simulink model "AC_DC_BUCK_2022b"  (R2022b)
settings: Solver=VariableStepAuto  StartTime=0.0  StopTime=3  RelTol=1e-3
libraries: spsSeriesRLCBranchLib x16, spsIdealSwitchLib x9, gmp_peripheral_utilities x6, spsVoltageMeasurementLib x6, spsSecondOrderFilterLib x5, spsControlledVoltageSourceLib x3, spsCurrentMeasurementLib x2, gmp_sil_core_pack x1, spspowerguiLib x1
(part 1 of 2)
settings Model: SimulationMode=accelerator  Creator=javnson  LastModifiedBy=javnson
settings DataIOCC: ReturnWorkspaceOutputs=off
settings OptimizationCC: ReuseModelBlockBuffer=on
settings RTWCC: GPUComputeCapability=5.0

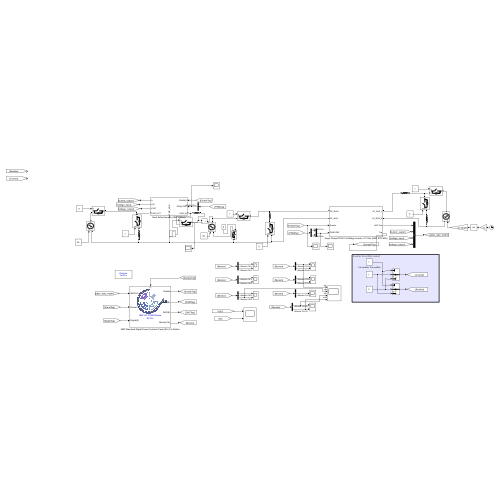
[thumbnail: Simulink's stored preview of the top-level diagram]
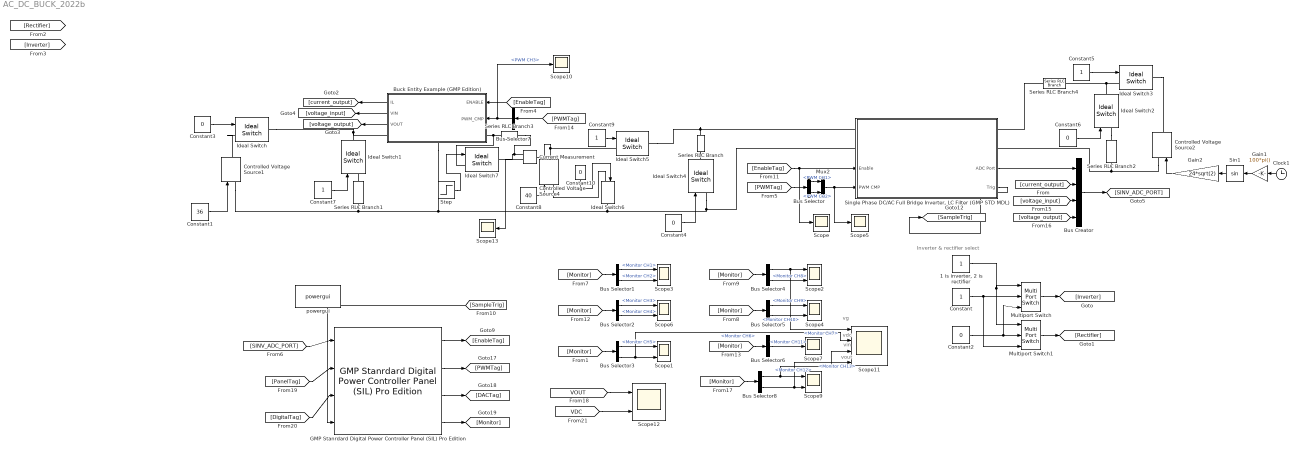
== system AC_DC_BUCK_2022b ==
  note: vout
  note: vin
  note: vg
  note: vdc
  note: Inverter & rectifier select
  "1 is inverter, 2 is rectifier" : Constant
  Buck Entity Example (GMP Edition) : Subsystem  mask{Cin=680e-6, Cout=680e-6, L=50e-6, RL=1e-3, RCin=0.1, RCout=100e-6, Cout2=680e-6, RCout2=1e-4, Voadc_bias=0, Voadc_fs=120, ADC_RES=16, Viadc_fs=120, Viadc_bias=0, Iladc_fs=60, Iadc_bias=30, fswitch=20e3, CMP_MAX=4200-1, DB_UP=100, DB_DW=100, Rds_on=0.02, Lon=0, Rd=0.01, Vf=0.3, Rs=1e5, Cs=inf}
      settings: PortSchema="{\"entries\":[{\"content\":{\"sides\":[{\"content\":{\"connectorIds\":[\"In1\",\"In2\",\"LConn1\"]},\"type\":\"ConnectorPlacement.EquallySpacedRectSide\",\"uuid\":\"3dc1f0aa-256b-4eee-9ab4-ff52cb056450\"},{\"content\":{\"connectorIds\":[\"Out1\",\"Out2\",\"Out3\",\"RConn1\"],\"side\":\"RIGHT\"},\"type\":\"ConnectorPlacement.EquallySpacedRectSide\",\"uuid\":\"c182f68c-961e-48e9-b450-8a2d07cca989\"},{\"content\":{\"connectorIds\":[],\"side\":\"TOP\"},\"type\":\"ConnectorPlacement.EquallySpacedRectSide\",\"uuid\":\"77cafdf0-ba99-4ec6-a003-27712a389068\"},{\"content\":{\"connectorIds\":[\"RConn2\"],\"side\":\"BOTTOM\"},\"type\":\"ConnectorPlacement.EquallySpacedRectSide\",\"uuid\":\"1cb5a4dc-5d4b-4bbe-a9bd-2c66268ddaed\"}]},\"type\":\"ConnectorPlacement.EquallySpacedConnector\",\"uuid\":\"ec8c1d3d-5436-4386-91dc-89cedd685bc0\"}],\"packageUris\":[\"http://schema.mathworks.com/mf0/Connector/R2020b\"],\"version\":\"1.0\"}"
      mask DialogControl Container4 Prompt: Main Circuit
      mask DialogControl Control2 Prompt: Input port Capacitor, unit F
      mask DialogControl Control3 Prompt: Ouput port Capacitor, unit F
      mask DialogControl Control4 Prompt: Filter Inductor, unit H
      mask DialogControl Container6 Prompt: Other Parameters
      mask DialogControl Control5 Prompt: Resistance of Inductor, unit Ohm
      mask DialogControl Control9 Prompt: Resistance of input Capacitor, unit Ohm
      mask DialogControl Control6 Prompt: Resistance of output Capacitor, unit Ohm
      mask DialogControl Control7 Prompt: Low resistance output Capacitor branch, Capacitor, unit F
      mask DialogControl Control8 Prompt: Low resistance output capacitor branch, resistance of capacitor, unit Ohm
      mask DialogControl Container5 Prompt: Sensor
      mask DialogControl Control15 Prompt: Output Voltage ADC, Bias Voltage, unit V
      mask DialogControl Control14 Prompt: Output Voltage ADC, Full Scale Voltage, unit V
      mask DialogControl Control10 Prompt: ADC resolution, bits
      mask DialogControl Control11 Prompt: Input Voltage ADC, Full Scale Voltage, unit V
      mask DialogControl Control12 Prompt: Input Voltage ADC, Bias Voltage, unit V
      mask DialogControl Control13 Prompt: Indctor Current ADC, Full Scale, unit A
      mask DialogControl Control16 Prompt: Inductor Current ADC, Bias Current, unit A
      mask DialogControl Container7 Prompt: PWM Modulator
      mask DialogControl Control17 Prompt: PWM frequency, unit Hz
      mask DialogControl Control18 Prompt: Full Scale PWM Compare value
      mask DialogControl Control19 Prompt: Deadband Setting
      mask DialogControl Container8 Prompt: MOSFET
      mask DialogControl Control20 Prompt: Rds(on), unit Ohm
      mask DialogControl Control21 Prompt: Internal diode inductance, unit H
      mask DialogControl Control22 Prompt: Internal diode resistance Rd, unit Ohm
      mask DialogControl Control23 Prompt: Internal diode forward voltage Vf, unit V
      mask DialogControl Control24 Prompt: Snubber resistance Rs, unit Ohm
      mask DialogControl Control25 Prompt: Snubber Capacitance Cs, unit F
  Bus Creator : BusCreator  Inputs=4
  Bus Selector : BusSelector  OutputSignals=PWM CH1,PWM CH2
  Bus Selector1 : BusSelector  OutputSignals=Monitor CH1,Monitor CH2
  Bus Selector2 : BusSelector  OutputSignals=Monitor CH3,Monitor CH4
  Bus Selector3 : BusSelector  OutputSignals=Monitor CH5,Monitor CH6
  Bus Selector4 : BusSelector  OutputSignals=Monitor CH7,Monitor CH8
  Bus Selector5 : BusSelector  OutputSignals=Monitor CH9,Monitor CH10
  Bus Selector6 : BusSelector  OutputSignals=Monitor CH11
  Bus Selector7 : BusSelector  OutputSignals=PWM CH3
  Bus Selector8 : BusSelector  OutputSignals=Monitor CH12,Monitor CH13
  Clock1 : Clock
  Constant{,5,7,9} (4 alike) : Constant
  Constant1 : Constant  Value=36
  Constant{2..4,6,10} (5 alike) : Constant  Value=0
  Constant8 : Constant  Value=40
  Controlled Voltage Source1 : spsControlledVoltageSourceLib/Controlled Voltage Source  Initialize=on  Source_Type=AC  Amplitude=0  Phase=0  Frequency=0  Measurements=None
  Controlled Voltage Source2 : spsControlledVoltageSourceLib/Controlled Voltage Source  Initialize=on  Source_Type=AC  Amplitude=0  Phase=0  Frequency=0  Measurements=None
  Controlled Voltage Source4 : spsControlledVoltageSourceLib/Controlled Voltage Source  Initialize=on  Source_Type=AC  Amplitude=0  Phase=0  Frequency=0  Measurements=None
  Current Measurement : spsCurrentMeasurementLib/Current Measurement  PhasorSimulation=off  OutputType=Complex  PSBequivalent=0
  GMP Stanrdard Digital Power Controller Panel (SIL) Pro Edition : gmp_sil_core_pack/GMP Stanrdard Digital Power Controller Panel (SIL) Pro Edition
      settings: SourceProductName=GMP SIL Core Utilities
  Gain1 : Gain  Gain=100*pi()
  Gain2 : Gain  Gain=24*sqrt(2)
  Ideal Switch{,1..7} (8 alike) : spsIdealSwitchLib/Ideal Switch  Ron=0.001  Lon=0  IC=0  Rs=1e5  Cs=inf  Measurements=off
  Multiport Switch : MultiPortSwitch  Inputs=2  SaturateOnIntegerOverflow=off  InputSameDT=off
  Multiport Switch1 : MultiPortSwitch  Inputs=2  SaturateOnIntegerOverflow=off  InputSameDT=off
  Mux2 : Mux  Inputs=2
  Scope{,5,7,10,13} (5 alike) : Scope
  Scope{1..4,6,9,12} (7 alike) : Scope  NumInputPorts=2
  Scope11 : Scope  NumInputPorts=4
  Series RLC Branch : spsSeriesRLCBranchLib/Series RLC Branch  LConnTagsString=__new0  RConnTagsString=__new0  BranchType=R  Resistance=100  Inductance=1e-3  SetiL0=off  InitialCurrent=0  Capacitance=1e-6  Setx0=off  InitialVoltage=0  Measurements=None
  Series RLC Branch1 : spsSeriesRLCBranchLib/Series RLC Branch  LConnTagsString=__new0  RConnTagsString=__new0  BranchType=R  Resistance=200  Inductance=1e-3  SetiL0=off  InitialCurrent=0  Capacitance=1e-6  Setx0=off  InitialVoltage=0  Measurements=None
  Series RLC Branch2 : spsSeriesRLCBranchLib/Series RLC Branch  LConnTagsString=__new0  RConnTagsString=__new0  BranchType=R  Resistance=18  Inductance=1e-3  SetiL0=off  InitialCurrent=0  Capacitance=1e-6  Setx0=off  InitialVoltage=0  Measurements=None
  Series RLC Branch3 : spsSeriesRLCBranchLib/Series RLC Branch  LConnTagsString=__new0  RConnTagsString=__new0  BranchType=R  Resistance=100  Inductance=1e-3  SetiL0=off  InitialCurrent=0  Capacitance=1e-6  Setx0=off  InitialVoltage=0  Measurements=None
  Series RLC Branch4 : spsSeriesRLCBranchLib/Series RLC Branch  LConnTagsString=__new0  RConnTagsString=__new0  BranchType=R  Resistance=2  Inductance=1e-3  SetiL0=off  InitialCurrent=0  Capacitance=1e-6  Setx0=off  InitialVoltage=0  Measurements=None
  Sin1 : Trigonometry
  "Single Phase DC/AC Full Bridge Inverter, LC Filter (GMP STD MDL)" : Subsystem  mask(Standard Single Phase DC/AC inverter / rectifier){R_mosfet_on=4.6e-3, Lon=0, Rd=0.01, Vf=0.5, Rs=1e5, Cs=inf, ACF_L=680e-6*2, ACF_L_ESR=0.05, ACF_C=10e-6, ACF_C_ESR=0.02, ACF_C_EPR=100e3, DC_CAP=680e-6, DC_CAP_ESR=0.05, DC_CAP_EPR=10e3, fswitch=20e3, CMP_MAX=4200-1, Deadband_Upper=80, Deadband_Lower=80, phase_shift=0, ADC_Resolution=12, DC_Voltage_Gain=2.2 / 202.2, DC_VOLTAGE_ADC_REFERENCE=2.5, DC_VOLTAGE_ADC_BIAS=0.9966, DC_VOLTAGE_ADC_CUT_FREQ=1.5e3, DC_BUS_CURRENT_SENSOR_R=0.005, DC_Current_Gain=20, DC_CURRENT_ADC_REFERENCE=2.5, DC_CURRENT_ADC_BIAS=0.9, DC_CURRENT_ADC_CUT_FREQ=1.5e3, AC_Voltage_Gain=2.2 / 202.2, AC_VOLTAGE_ADC_REFERENCE=2.5, AC_VOLTAGE_ADC_BIAS=0.9966, AC_VOLTAGE_ADC_CUT_FREQ=1.5e3, AC_Current_Gain=0.005 * 20, AC_CURRENT_ADC_REFERENCE=2.5, AC_CURRENT_ADC_BIAS=0.9, AC_CURRENT_ADC_INIT=0, CAP_CURRENT_SENSOR_R=0.005, CAP_Current_Gain=20, CAP_CURRENT_ADC_REFERENCE=2.5, CAP_CURRENT_ADC_BIAS=0.9, CAP_CURRENT_ADC_CUT_FREQ=1.5e3, GRID_CURRENT_SENSOR_R=0.005, Grid_Current_Gain=20, GRID_CURRENT_ADC_REFERENCE=2.5, GRID_CURRENT_ADC_BIAS=0.9, GRID_CURRENT_ADC_CUT_FREQ=1.5e3}
      mask prompts: ADC_Resolution "ADC_BIT:"; DC_Voltage_Gain "ADC_GAIN:"; DC_VOLTAGE_ADC_REFERENCE "ADC_REFERENCE:"; DC_VOLTAGE_ADC_BIAS "ADC_BIAS:"; DC_VOLTAGE_ADC_CUT_FREQ "cut_frequency:"; DC_Current_Gain "ADC_GAIN:"; DC_CURRENT_ADC_REFERENCE "ADC_REFERENCE:"; DC_CURRENT_ADC_BIAS "ADC_BIAS:"; DC_CURRENT_ADC_CUT_FREQ "ADC_FILTER:"; AC_Voltage_Gain "ADC_GAIN:"; AC_VOLTAGE_ADC_REFERENCE "ADC_REFERENCE:"; AC_VOLTAGE_ADC_BIAS "ADC_BIAS:"; AC_VOLTAGE_ADC_CUT_FREQ "cut_frequency:"; AC_Current_Gain "ADC_GAIN:"; AC_CURRENT_ADC_REFERENCE "ADC_REFERENCE:"; AC_CURRENT_ADC_BIAS "ADC_BIAS:"; AC_CURRENT_ADC_INIT "ADC_INIT:"; CAP_CURRENT_SENSOR_R "CAP_BUS_CURRENT_SENSOR_R:"; CAP_Current_Gain "ADC_GAIN:"; CAP_CURRENT_ADC_REFERENCE "ADC_REFERENCE:"; CAP_CURRENT_ADC_BIAS "ADC_BIAS:"; CAP_CURRENT_ADC_CUT_FREQ "ADC_FILTER:"; GRID_CURRENT_SENSOR_R "DC_BUS_CURRENT_SENSOR_R:"; Grid_Current_Gain "ADC_GAIN:"; GRID_CURRENT_ADC_REFERENCE "ADC_REFERENCE:"; GRID_CURRENT_ADC_BIAS "ADC_BIAS:"; GRID_CURRENT_ADC_CUT_FREQ "ADC_FILTER:"
      mask help: This module takes the inverter direction as the positive direction.
      settings: PortSchema="{\"entries\":[{\"content\":{\"sides\":[{\"content\":{\"connectorIds\":[\"LConn1\",\"LConn2\",\"In1\",\"In2\"]},\"type\":\"ConnectorPlacement.EquallySpacedRectSide\",\"uuid\":\"0e3e6e75-5e1a-455b-8a22-c69d0a4261ca\"},{\"content\":{\"connectorIds\":[\"RConn1\",\"RConn2\",\"Out1\",\"Out2\"],\"side\":\"RIGHT\"},\"type\":\"ConnectorPlacement.EquallySpacedRectSide\",\"uuid\":\"20326781-9238-4fea-80fd-ba96906d5d3f\"},{\"content\":{\"side\":\"TOP\"},\"type\":\"ConnectorPlacement.EquallySpacedRectSide\",\"uuid\":\"9e3289d3-0bee-4337-807b-c293a46cda9c\"}]},\"type\":\"ConnectorPlacement.EquallySpacedConnector\",\"uuid\":\"56bb35ad-d602-4874-b9bf-b95a81ef662c\"}],\"packageUris\":[\"http://schema.mathworks.com/mf0/Connector/R2020b\"],\"version\":\"1.0\"}"
      mask DialogControl ParameterGroupVar Prompt: 参数
      mask DialogControl Container4 Prompt: Component Parameters
      mask DialogControl Container7 Prompt: MOSFET
      mask DialogControl Control2 Prompt: Rds(on), unit Ohm
      mask DialogControl Control3 Prompt: Internal diode inducctance, unit H
      mask DialogControl Control4 Prompt: Internal diode resistance Rd, unit Ohm
      mask DialogControl Control5 Prompt: Internal diode forward voltage Vf, unit V
      mask DialogControl Control6 Prompt: Snubber resistance Rs, unit ohm
      mask DialogControl Control7 Prompt: Snubber Capacitance Cs, unit F
      mask DialogControl Container8 Prompt: LC Filter
      mask DialogControl Container20 Prompt: Filter Inductor
      mask DialogControl Control8 Prompt: AC Bus Filter Inductor (H)
      mask DialogControl Control42 Prompt: AC Bus Filter Inductor, ESR (Ohm)
      mask DialogControl Container21 Prompt: Filter Capcitor
      mask DialogControl Control43 Prompt: AC Bus Filter Capacitor (F)
      mask DialogControl Control44 Prompt: AC Bus Filter Capacitor, ESR (Ohm)
      mask DialogControl Control45 Prompt: AC Bus Filter Capacitor, EPR (Ohm)
      mask DialogControl Container22 Prompt: DC Bus Capacitor
      mask DialogControl Control46 Prompt: DC Bus Capacitor (F)
      mask DialogControl Control47 Prompt: DC Bus Capacitor, ESR (Ohm)
      mask DialogControl Control48 Prompt: DC Bus Capacitor, EPR (Ohm)
      mask DialogControl Container5 Prompt: PWM Parameers
      mask DialogControl Control9 Prompt: PWM Frequency (Hz):
      mask DialogControl Control10 Prompt: Full Scale PWM Compare value:
      mask DialogControl Control11 Prompt: (whole period is 2 * CMP_MAX ticks)
      mask DialogControl Control12 Prompt: Deadband Range Set (CMP Value):
      mask DialogControl Control13 Prompt: Single side deadband time: DEADBAND_CMP/2/CMP_MAX/fswitch
      mask DialogControl Control14 Prompt: Initial Phase Shift, unit rad
      mask DialogControl Container6 Prompt: ADC Parameters
      mask DialogControl Container14 Prompt: ADC Device
      mask DialogControl Control15 Prompt: ADC resolution:
      mask DialogControl Container15 Prompt: DC Side Voltage Sensor
      mask DialogControl Control16 Prompt: ADC Voltage Gain (Scale Factor):
      mask DialogControl Control17 Prompt: ADC reference Voltage(V)
      mask DialogControl Control18 Prompt: ADC Bias Voltage(V)
      mask DialogControl Control19 Prompt: Voltage Filter cut frequency (Hz):
      mask DialogControl Control20 Prompt: Generally, this value less than switch frequency / 10, greater than motor normal frequency * 3
      mask DialogControl Container16 Prompt: DC Side Current Sensor
      mask DialogControl Control26 Prompt: DC Bus Current Sensor Resistance
      mask DialogControl Control34 Prompt: ADC Current Gain (Scale Factor):
      mask DialogControl Control27 Prompt: ADC reference Voltage(V), ADC full scale current (when gain = 1)
      mask DialogControl Control28 Prompt: ADC Bias Current(A)
      mask DialogControl Control35 Prompt: Voltage Filter cut frequency (Hz):
      mask DialogControl Control36 Prompt: Generally, this value less than switch frequency / 10, greater than motor normal frequency * 3
      mask DialogControl Container17 Prompt: AC Side Voltage Sensor
      mask DialogControl Control16_copy Prompt: ADC Voltage Gain (Scale Factor):
      mask DialogControl Control17_copy Prompt: ADC reference Voltage(V)
      mask DialogControl Control18_copy Prompt: ADC Bias Voltage(V)
      mask DialogControl Control19_copy Prompt: Voltage Filter cut frequency (Hz):
      mask DialogControl Control20_copy Prompt: Generally, this value less than switch frequency / 10, greater than motor normal frequency * 3
      mask DialogControl Container18 Prompt: AC Side Current Sensor
      mask DialogControl Control26_copy Prompt: ADC Current Gain (Scale Factor):
      mask DialogControl Control27_copy Prompt: ADC reference Current(A), ADC full scale current (when gain = 1)
      mask DialogControl Control28_copy Prompt: ADC Bias Current(A)
      mask DialogControl Control29_copy Prompt: ADC initial Current Output(A)
      mask DialogControl Container19 Prompt: Capcitor Current Sensor
      mask DialogControl Control26_copy_copy Prompt: Filter Capacitor Current Sensor Resistance
      mask DialogControl Control34_copy Prompt: ADC Current Gain (Scale Factor):
      mask DialogControl Control27_copy_copy Prompt: ADC reference Voltage(V), ADC full scale current (when gain = 1)
      mask DialogControl Control28_copy_copy Prompt: ADC Bias Current(V)
      mask DialogControl Control35_copy Prompt: Voltage Filter cut frequency (Hz):
      mask DialogControl Control36_copy Prompt: Generally, this value less than switch frequency / 10, greater than motor normal frequency * 3
      mask DialogControl Container23 Prompt: Grid Current Sensor
      mask DialogControl Control26_copy_copy_copy Prompt: Grid Bus Current Sensor Resistance
      mask DialogControl Control34_copy_copy Prompt: ADC Current Gain (Scale Factor):
      mask DialogControl Control27_copy_copy_copy Prompt: ADC reference Voltage(V), ADC full scale current (when gain = 1)
      mask DialogControl Control28_copy_copy_copy Prompt: ADC Bias Current(V)
      mask DialogControl Control35_copy_copy Prompt: Voltage Filter cut frequency (Hz):
      mask DialogControl Control36_copy_copy Prompt: Generally, this value less than switch frequency / 10, greater than motor normal frequency * 3
  Step : Step  Before=1  SampleTime=0
  powergui : spspowerguiLib/powergui  Priority=1  SimulationMode=Discrete  SampleTime=1e-6  frequency=60  Iterations=50  frequencyindice=0  Pbase=100e6  ErrMax=1e-4  UnitsV=kV  UnitsW=MW  buscounter=0  FunctionMessages=off  echomessages=off  EnableUseOfTLC=off  CurrentSourceSwitches=off  DisableSnubberDevices=off  DisableRonSwitches=off  DisableVfSwitches=off  DisplayEquations=off  AutomaticDiscreteSolvers=off  SolverType=Tustin/Backward Euler (TBE)  Interpol=off  ExternalGateDelay=off  methode=off  Ts=100  x0status=blocks  SPID=on  SwTol=0  HookPort=off  NonlinearTolerance=1e-4  nMaxIteration=100  ContinueOnMaxIteration=off  RestoreLinks=warning  ResistiveCurrentMeasurement=off  Frange=[0:2:500]  Ylog=off  Xlog=on  ShowGrid=off  save=off  variable=ZData  structure=0  ZoomFFT=off  StartTime=0.0  cycles=1  DisplayStyle=1  fundamental=60  FreqAxis=off  MaxFrequency=1000  frequencyindicesteady=1  RmsSteady=1  display=off
  wires:
  Constant1/1 -> Controlled Voltage Source1/1
  [EnableTag] -> Scope/1, "Single Phase DC/AC Full Bridge Inverter, LC Filter (GMP STD MDL)"/1(Enable)
  "Single Phase DC/AC Full Bridge Inverter, LC Filter (GMP STD MDL)"/2(Trig) -> [SampleTrig]
  Gain1/1 -> Sin1/1
  Clock1/1 -> Gain1/1
  Sin1/1 -> Gain2/1
  Gain2/1 -> Controlled Voltage Source2/1
  [SampleTrig] -> GMP Stanrdard Digital Power Controller Panel (SIL) Pro Edition/4
  GMP Stanrdard Digital Power Controller Panel (SIL) Pro Edition/1 -> [EnableTag]
  GMP Stanrdard Digital Power Controller Panel (SIL) Pro Edition/2 -> [PWMTag]
  GMP Stanrdard Digital Power Controller Panel (SIL) Pro Edition/3 -> [DACTag]
  GMP Stanrdard Digital Power Controller Panel (SIL) Pro Edition/4 -> [Monitor]
  [SINV_ADC_PORT] -> GMP Stanrdard Digital Power Controller Panel (SIL) Pro Edition/1
  [PanelTag] -> GMP Stanrdard Digital Power Controller Panel (SIL) Pro Edition/2
  [DigitalTag] -> GMP Stanrdard Digital Power Controller Panel (SIL) Pro Edition/3
  [PWMTag] -> Bus Selector/1
  Bus Selector/1 -> Mux2/1  "<PWM CH1>"
  Bus Selector/2 -> Mux2/2  "<PWM CH2>"
  Mux2/1 -> Scope5/1, "Single Phase DC/AC Full Bridge Inverter, LC Filter (GMP STD MDL)"/2(PWM CMP)
  [Monitor] -> Bus Selector1/1
  Bus Selector1/1 -> Scope3/1  "<Monitor CH1>"
  Bus Selector1/2 -> Scope3/2  "<Monitor CH2>"
  [Monitor] -> Bus Selector2/1
  Bus Selector2/1 -> Scope6/1  "<Monitor CH3>"
  Bus Selector2/2 -> Scope6/2  "<Monitor CH4>"
  Bus Selector3/2 -> Scope11/2, Scope1/2  "<Monitor CH6>"
  Bus Selector3/1 -> Scope1/1  "<Monitor CH5>"
  [Monitor] -> Bus Selector3/1
  "1 is inverter, 2 is rectifier"/1 -> Multiport Switch/1, Multiport Switch1/1
  Constant/1 -> Multiport Switch/2, Multiport Switch1/3
  Constant2/1 -> Multiport Switch1/2, Multiport Switch/3
  Multiport Switch/1 -> [Inverter]
  Multiport Switch1/1 -> [Rectifier]
  Bus Selector5/2 -> Scope4/2  "<Monitor CH10>"
  Bus Selector5/1 -> Scope4/1  "<Monitor CH9>"
  [Monitor] -> Bus Selector5/1
  [Monitor] -> Bus Selector4/1
  Bus Selector4/1 -> Scope11/1, Scope2/1  "<Monitor CH7>"
  Bus Selector4/2 -> Scope2/2  "<Monitor CH8>"
  [Monitor] -> Bus Selector6/1
  Bus Selector6/1 -> Scope7/1  "<Monitor CH11>"
  [EnableTag] -> Buck Entity Example (GMP Edition)/1(ENABLE)
  Bus Selector7/1 -> Scope10/1, Buck Entity Example (GMP Edition)/2(PWM_CMP)  "<PWM CH3>"
  Constant3/1 -> Ideal Switch/1
  Constant5/1 -> Ideal Switch3/1
  Constant6/1 -> Ideal Switch2/1
  Buck Entity Example (GMP Edition)/2(VIN) -> [voltage_input]
  Buck Entity Example (GMP Edition)/1(IL) -> [current_output]
  Buck Entity Example (GMP Edition)/3(VOUT) -> [voltage_output]
  "Single Phase DC/AC Full Bridge Inverter, LC Filter (GMP STD MDL)"/1(ADC Port) -> Bus Creator/1
  [current_output] -> Bus Creator/2
  [voltage_input] -> Bus Creator/3
  [voltage_output] -> Bus Creator/4
  Bus Creator/1 -> [SINV_ADC_PORT]
  [Monitor] -> Bus Selector8/1
  Bus Selector8/1 -> Scope11/3, Scope9/1  "<Monitor CH12>"
  [PWMTag] -> Bus Selector7/1
  Constant8/1 -> Controlled Voltage Source4/1
  Constant9/1 -> Ideal Switch5/1
  Bus Selector8/2 -> Scope11/4, Scope9/2  "<Monitor CH13>"
  Constant10/1 -> Ideal Switch6/1
  [VOUT] -> Scope12/1
  [VDC] -> Scope12/2
  Constant4/1 -> Ideal Switch4/1
  Current Measurement/1 -> Scope13/1
  Constant7/1 -> Ideal Switch1/1
  Step/1 -> Ideal Switch7/1
  connections:
  Controlled Voltage Source1/LConn1 -- Buck Entity Example (GMP Edition)/RConn2 -- Ideal Switch4/LConn1 -- "Single Phase DC/AC Full Bridge Inverter, LC Filter (GMP STD MDL)"/LConn2 -- Ideal Switch6/RConn1 -- Series RLC Branch1/RConn1
  Series RLC Branch4/RConn1 -- "Single Phase DC/AC Full Bridge Inverter, LC Filter (GMP STD MDL)"/RConn1
  Controlled Voltage Source2/LConn1 -- Series RLC Branch2/RConn1 -- "Single Phase DC/AC Full Bridge Inverter, LC Filter (GMP STD MDL)"/RConn2
  Ideal Switch/LConn1 -- Controlled Voltage Source1/RConn1
  Series RLC Branch1/LConn1 -- Ideal Switch1/LConn1
  Ideal Switch2/LConn1 -- Series RLC Branch2/LConn1
  Ideal Switch3/RConn1 -- Controlled Voltage Source2/RConn1
  Series RLC Branch/LConn1 -- "Single Phase DC/AC Full Bridge Inverter, LC Filter (GMP STD MDL)"/LConn1 -- Ideal Switch5/RConn1
  Ideal Switch2/RConn1 -- Series RLC Branch4/LConn1 -- Ideal Switch3/LConn1
  Buck Entity Example (GMP Edition)/RConn1 -- Ideal Switch/RConn1 -- Ideal Switch1/RConn1
  Series RLC Branch/RConn1 -- Ideal Switch4/RConn1
  Controlled Voltage Source4/RConn1 -- Current Measurement/LConn1 -- Ideal Switch5/LConn1
  Controlled Voltage Source4/LConn1 -- Ideal Switch6/LConn1
  Series RLC Branch3/RConn1 -- Ideal Switch7/LConn1 -- Buck Entity Example (GMP Edition)/LConn1
  Series RLC Branch3/LConn1 -- Ideal Switch7/RConn1 -- Current Measurement/RConn1

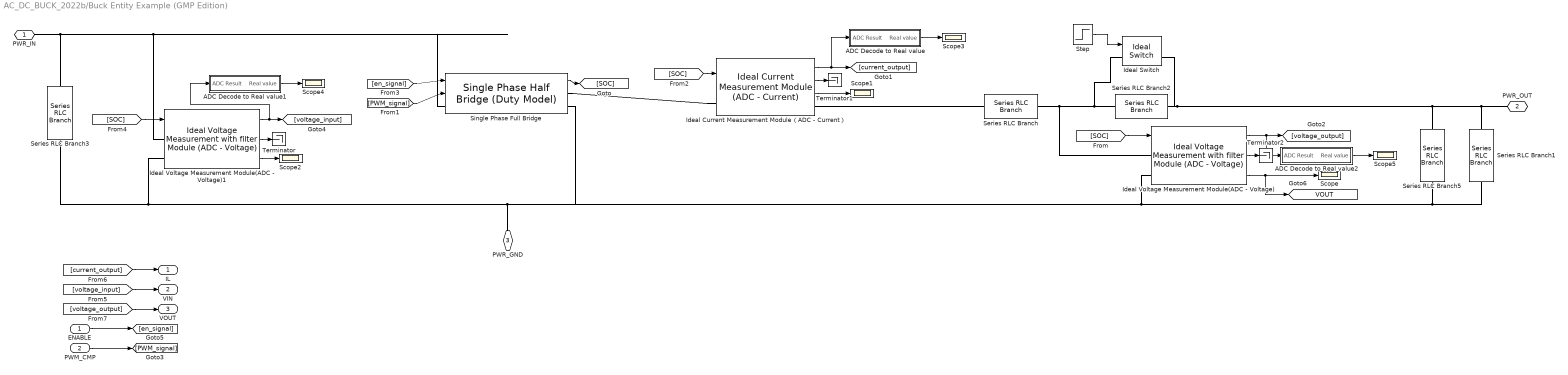
== system AC_DC_BUCK_2022b/Buck Entity Example (GMP Edition) ==
  ENABLE : Inport
  PWM_CMP : Inport  Port=2
  ADC Decode to Real value : Subsystem  mask{ADC_GAIN=1, ADC_BIT=16, ADC_REF=60, ADC_BIAS=30}
      settings: CopyFcn=set_param(gcbh,'LinkStatus','none');
      mask DialogControl DescGroupVar Prompt: ADC Decoder
      mask DialogControl DescTextVar Prompt: GMP CTL Simulink Utilities: virtual peripherals
      mask DialogControl Control2 Prompt: Transfer adc sample result to real value.
      mask DialogControl ParameterGroupVar Prompt: 参数
      mask DialogControl Control3 Prompt: ADC Voltage Gain (Scale Factor):
      mask DialogControl Control4 Prompt: ADC resolution:
      mask DialogControl Control5 Prompt: ADC reference Voltage (V), when ADC_GAIN=1, ADC_REF = ADC full scale
      mask DialogControl Control6 Prompt: ADC Bias Voltage(V)
  ADC Decode to Real value1 : Subsystem  mask{ADC_GAIN=1, ADC_BIT=16, ADC_REF=120, ADC_BIAS=0}
      settings: CopyFcn=set_param(gcbh,'LinkStatus','none');
      mask DialogControl DescGroupVar Prompt: ADC Decoder
      mask DialogControl DescTextVar Prompt: GMP CTL Simulink Utilities: virtual peripherals
      mask DialogControl Control2 Prompt: Transfer adc sample result to real value.
      mask DialogControl ParameterGroupVar Prompt: 参数
      mask DialogControl Control3 Prompt: ADC Voltage Gain (Scale Factor):
      mask DialogControl Control4 Prompt: ADC resolution:
      mask DialogControl Control5 Prompt: ADC reference Voltage (V), when ADC_GAIN=1, ADC_REF = ADC full scale
      mask DialogControl Control6 Prompt: ADC Bias Voltage(V)
  ADC Decode to Real value2 : Subsystem  mask{ADC_GAIN=1, ADC_BIT=16, ADC_REF=120, ADC_BIAS=0}
      settings: CopyFcn=set_param(gcbh,'LinkStatus','none');
      mask DialogControl DescGroupVar Prompt: ADC Decoder
      mask DialogControl DescTextVar Prompt: GMP CTL Simulink Utilities: virtual peripherals
      mask DialogControl Control2 Prompt: Transfer adc sample result to real value.
      mask DialogControl ParameterGroupVar Prompt: 参数
      mask DialogControl Control3 Prompt: ADC Voltage Gain (Scale Factor):
      mask DialogControl Control4 Prompt: ADC resolution:
      mask DialogControl Control5 Prompt: ADC reference Voltage (V), when ADC_GAIN=1, ADC_REF = ADC full scale
      mask DialogControl Control6 Prompt: ADC Bias Voltage(V)
  Ideal Current Measurement Module（ADC - Current） : gmp_peripheral_utilities/Ideal Current Measurement Module (ADC - Current)  ADC_GAIN=0.005*20  ADC_BIT=12  ADC_REFERENCE=2.5  ADC_BIAS=0.9  ADC_INIT=0
      settings: SourceProductName=Virtual Peripheral Utilities
  Ideal Switch : spsIdealSwitchLib/Ideal Switch  Ron=0.001  Lon=0  IC=0  Rs=1e5  Cs=inf  Measurements=on
  Ideal Voltage Measurement Module(ADC - Voltage) : gmp_peripheral_utilities/Ideal Voltage Measurement with filter Module (ADC - Voltage)  ADC_GAIN=0.0109  ADC_BIT=12  ADC_REFERENCE=2.5  ADC_BIAS=0.9966  ADC_INIT=0  cut_frequency=500
      settings: SourceProductName=Virtual Peripheral Utilities
  Ideal Voltage Measurement Module(ADC - Voltage)1 : gmp_peripheral_utilities/Ideal Voltage Measurement with filter Module (ADC - Voltage)  ADC_GAIN=0.0109  ADC_BIT=12  ADC_REFERENCE=2.5  ADC_BIAS=0.9966  ADC_INIT=0  cut_frequency=500
      settings: SourceProductName=Virtual Peripheral Utilities
  Scope{,1..5} (6 alike) : Scope
  Series RLC Branch : spsSeriesRLCBranchLib/Series RLC Branch  LConnTagsString=__new0  RConnTagsString=__new0  BranchType=RL  Resistance=RL  Inductance=L  SetiL0=off  InitialCurrent=0  Capacitance=1e-6  Setx0=off  InitialVoltage=0  Measurements=None
  Series RLC Branch1 : spsSeriesRLCBranchLib/Series RLC Branch  LConnTagsString=__new0  RConnTagsString=__new0  BranchType=RC  Resistance=RCout2  Inductance=50e-6  SetiL0=off  InitialCurrent=0  Capacitance=Cout2  Setx0=off  InitialVoltage=0  Measurements=None
  Series RLC Branch2 : spsSeriesRLCBranchLib/Series RLC Branch  LConnTagsString=__new0  RConnTagsString=__new0  BranchType=R  Resistance=50  Inductance=1e-3  SetiL0=off  InitialCurrent=0  Capacitance=1e-6  Setx0=off  InitialVoltage=0  Measurements=None
  Series RLC Branch3 : spsSeriesRLCBranchLib/Series RLC Branch  LConnTagsString=__new0  RConnTagsString=__new0  BranchType=RC  Resistance=RCin  Inductance=50e-6  SetiL0=off  InitialCurrent=0  Capacitance=Cin  Setx0=off  InitialVoltage=0  Measurements=None
  Series RLC Branch5 : spsSeriesRLCBranchLib/Series RLC Branch  LConnTagsString=__new0  RConnTagsString=__new0  BranchType=RC  Resistance=RCout  Inductance=50e-6  SetiL0=off  InitialCurrent=0  Capacitance=Cout  Setx0=off  InitialVoltage=0  Measurements=None
  Single Phase Full Bridge : gmp_peripheral_utilities/Single Phase Half Bridge (Duty Model)  fswitch=fswitch  CMP_MAX=CMP_MAX  Deadband_Upper=DB_UP  Deadband_Lower=DB_DW  Deadband_us=NaN  phase_shift=0  R_mosfet_on=Rds_on  Lon=Lon  Rd=Rd  Vf=Vf  Rs=Rs  Cs=Cs
      settings: SourceProductName=Virtual Peripheral Utilities
  Step : Step  Before=1  SampleTime=0
  Terminator : Terminator
  Terminator1 : Terminator
  Terminator2 : Terminator
  PWR_IN : PMIOPort  Side=Left
  PWR_OUT : PMIOPort  Port=2  Side=Right
  PWR_GND : PMIOPort  Port=3  Side=Right
  IL : Outport
  VIN : Outport  Port=2
  VOUT : Outport  Port=3
  tag scope: VOUT=global
  wires:
  [PWM_signal] -> Single Phase Full Bridge/2
  [SOC] -> Ideal Current Measurement Module（ADC - Current）/1
  Ideal Current Measurement Module（ADC - Current）/1 -> ADC Decode to Real value/1(ADC Result), [current_output]
  Ideal Voltage Measurement Module(ADC - Voltage)1/1 -> ADC Decode to Real value1/1(ADC Result), [voltage_input]
  Ideal Voltage Measurement Module(ADC - Voltage)/3 -> [VOUT], Scope/1
  Ideal Voltage Measurement Module(ADC - Voltage)/1 -> ADC Decode to Real value2/1(ADC Result), [voltage_output]
  [voltage_output] -> VOUT/1
  ENABLE/1 -> [en_signal]
  Ideal Current Measurement Module（ADC - Current）/3 -> Scope1/1
  Ideal Voltage Measurement Module(ADC - Voltage)1/3 -> Scope2/1
  [SOC] -> Ideal Voltage Measurement Module(ADC - Voltage)1/1
  Ideal Current Measurement Module（ADC - Current）/2 -> Terminator1/1
  [SOC] -> Ideal Voltage Measurement Module(ADC - Voltage)/1
  Single Phase Full Bridge/1 -> [SOC]
  PWM_CMP/1 -> [PWM_signal]
  ADC Decode to Real value2/1(Real value) -> Scope5/1
  [en_signal] -> Single Phase Full Bridge/1
  ADC Decode to Real value/1(Real value) -> Scope3/1
  ADC Decode to Real value1/1(Real value) -> Scope4/1
  Ideal Voltage Measurement Module(ADC - Voltage)/2 -> Terminator2/1
  Ideal Voltage Measurement Module(ADC - Voltage)1/2 -> Terminator/1
  [current_output] -> IL/1
  [voltage_input] -> VIN/1
  Step/1 -> Ideal Switch/1
  connections:
  Ideal Current Measurement Module（ADC - Current）/RConn1 -- Series RLC Branch/LConn1
  Series RLC Branch3/LConn1 -- PWR_IN/RConn1 -- Ideal Voltage Measurement Module(ADC - Voltage)1/LConn1 -- Single Phase Full Bridge/LConn1
  Ideal Current Measurement Module（ADC - Current）/LConn1 -- Single Phase Full Bridge/RConn1
  Series RLC Branch1/LConn1 -- PWR_OUT/RConn1 -- Ideal Switch/RConn1 -- Series RLC Branch2/RConn1 -- Series RLC Branch5/LConn1
  Ideal Voltage Measurement Module(ADC - Voltage)1/LConn2 -- PWR_GND/RConn1 -- Series RLC Branch1/RConn1 -- Series RLC Branch5/RConn1 -- Ideal Voltage Measurement Module(ADC - Voltage)/LConn2 -- Single Phase Full Bridge/RConn2 -- Series RLC Branch3/RConn1
  Series RLC Branch2/LConn1 -- Ideal Voltage Measurement Module(ADC - Voltage)/LConn1 -- Series RLC Branch/RConn1 -- Ideal Switch/LConn1

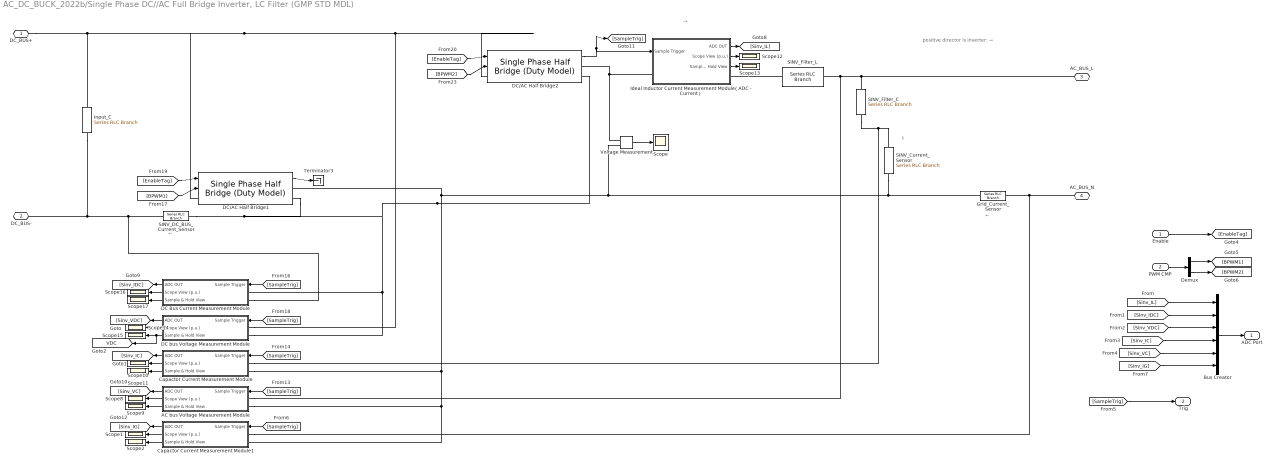
== system AC_DC_BUCK_2022b/Single Phase DC//AC Full Bridge Inverter, LC Filter (GMP STD MDL) ==
  note: ↓
  note: ←
  note: positive director is inverter: →
  note: ←
  note: →
  Enable : Inport
  PWM CMP : Inport  Port=2
  AC bus Voltage Measurement Module : Subsystem  AncestorBlock=peripheral_utilities/Ideal Voltage Measurement with filter Module(ADC - Voltage)  mask{ADC_GAIN=AC_Voltage_Gain, ADC_BIT=ADC_Resolution, ADC_REFERENCE=AC_VOLTAGE_ADC_REFERENCE, ADC_BIAS=AC_VOLTAGE_ADC_BIAS, ADC_INIT=0, cut_frequency=AC_VOLTAGE_ADC_CUT_FREQ}
      mask DialogControl DescGroupVar Prompt: Voltage Sample ADC Model
      mask DialogControl DescTextVar Prompt: This is a ideal Voltage Measurement Module.
      mask DialogControl Control2 Prompt: ADC(p.u.) = (real_voltage * ADC_GAIN + ADC_BIAS)/ADC_REFERENCE
      mask DialogControl Control11 Prompt: GMP CTL Simulink Utilities: virtual peripherals
      mask DialogControl ParameterGroupVar Prompt: Parameters:
      mask DialogControl Control4 Prompt: ADC Voltage Gain (Scale Factor):
      mask DialogControl Control5 Prompt: ADC resolution:
      mask DialogControl Control6 Prompt: ADC reference Voltage(V)
      mask DialogControl Control8 Prompt: ADC Bias Voltage(V)
      mask DialogControl Control7 Prompt: ADC Initial Voltage Output (V):
      mask DialogControl Control9 Prompt: Voltage Filter cut frequency (Hz):
      mask DialogControl Control10 Prompt: Generally, this value less than switch frequency / 10, greater than motor normal frequency * 3
  Bus Creator : BusCreator  Inputs=6
  Capactor Current Measurement Module : Subsystem  AncestorBlock=peripheral_utilities/Ideal Voltage Measurement with filter Module(ADC - Voltage)  mask{ADC_GAIN=CAP_Current_Gain, ADC_BIT=ADC_Resolution, ADC_REFERENCE=CAP_CURRENT_ADC_REFERENCE, ADC_BIAS=CAP_CURRENT_ADC_BIAS, ADC_INIT=0, cut_frequency=CAP_CURRENT_ADC_CUT_FREQ}
      mask DialogControl DescGroupVar Prompt: Voltage Sample ADC Model
      mask DialogControl DescTextVar Prompt: This is a ideal Voltage Measurement Module.
      mask DialogControl Control2 Prompt: ADC(p.u.) = (real_voltage * ADC_GAIN + ADC_BIAS)/ADC_REFERENCE
      mask DialogControl Control11 Prompt: GMP CTL Simulink Utilities: virtual peripherals
      mask DialogControl ParameterGroupVar Prompt: Parameters:
      mask DialogControl Control4 Prompt: ADC Voltage Gain (Scale Factor):
      mask DialogControl Control5 Prompt: ADC resolution:
      mask DialogControl Control6 Prompt: ADC reference Voltage(V)
      mask DialogControl Control8 Prompt: ADC Bias Voltage(V)
      mask DialogControl Control7 Prompt: ADC Initial Voltage Output (V):
      mask DialogControl Control9 Prompt: Voltage Filter cut frequency (Hz):
      mask DialogControl Control10 Prompt: Generally, this value less than switch frequency / 10, greater than motor normal frequency * 3
  Capactor Current Measurement Module1 : Subsystem  AncestorBlock=peripheral_utilities/Ideal Voltage Measurement with filter Module(ADC - Voltage)  mask{ADC_GAIN=Grid_Current_Gain, ADC_BIT=ADC_Resolution, ADC_REFERENCE=GRID_CURRENT_ADC_REFERENCE, ADC_BIAS=GRID_CURRENT_ADC_BIAS, ADC_INIT=0, cut_frequency=GRID_CURRENT_ADC_CUT_FREQ}
      mask DialogControl DescGroupVar Prompt: Voltage Sample ADC Model
      mask DialogControl DescTextVar Prompt: This is a ideal Voltage Measurement Module.
      mask DialogControl Control2 Prompt: ADC(p.u.) = (real_voltage * ADC_GAIN + ADC_BIAS)/ADC_REFERENCE
      mask DialogControl Control11 Prompt: GMP CTL Simulink Utilities: virtual peripherals
      mask DialogControl ParameterGroupVar Prompt: Parameters:
      mask DialogControl Control4 Prompt: ADC Voltage Gain (Scale Factor):
      mask DialogControl Control5 Prompt: ADC resolution:
      mask DialogControl Control6 Prompt: ADC reference Voltage(V)
      mask DialogControl Control8 Prompt: ADC Bias Voltage(V)
      mask DialogControl Control7 Prompt: ADC Initial Voltage Output (V):
      mask DialogControl Control9 Prompt: Voltage Filter cut frequency (Hz):
      mask DialogControl Control10 Prompt: Generally, this value less than switch frequency / 10, greater than motor normal frequency * 3
  DC Bus Current Measurement Module : Subsystem  AncestorBlock=peripheral_utilities/Ideal Voltage Measurement with filter Module(ADC - Voltage)  mask{ADC_GAIN=DC_Current_Gain, ADC_BIT=ADC_Resolution, ADC_REFERENCE=DC_CURRENT_ADC_REFERENCE, ADC_BIAS=DC_CURRENT_ADC_BIAS, ADC_INIT=0, cut_frequency=DC_CURRENT_ADC_CUT_FREQ}
      mask DialogControl DescGroupVar Prompt: Voltage Sample ADC Model
      mask DialogControl DescTextVar Prompt: This is a ideal Voltage Measurement Module.
      mask DialogControl Control2 Prompt: ADC(p.u.) = (real_voltage * ADC_GAIN + ADC_BIAS)/ADC_REFERENCE
      mask DialogControl Control11 Prompt: GMP CTL Simulink Utilities: virtual peripherals
      mask DialogControl ParameterGroupVar Prompt: Parameters:
      mask DialogControl Control4 Prompt: ADC Voltage Gain (Scale Factor):
      mask DialogControl Control5 Prompt: ADC resolution:
      mask DialogControl Control6 Prompt: ADC reference Voltage(V)
      mask DialogControl Control8 Prompt: ADC Bias Voltage(V)
      mask DialogControl Control7 Prompt: ADC Initial Voltage Output (V):
      mask DialogControl Control9 Prompt: Voltage Filter cut frequency (Hz):
      mask DialogControl Control10 Prompt: Generally, this value less than switch frequency / 10, greater than motor normal frequency * 3
  DC bus Voltage Measurement Module : Subsystem  AncestorBlock=peripheral_utilities/Ideal Voltage Measurement with filter Module(ADC - Voltage)  mask{ADC_GAIN=DC_Voltage_Gain, ADC_BIT=ADC_Resolution, ADC_REFERENCE=DC_VOLTAGE_ADC_REFERENCE, ADC_BIAS=DC_VOLTAGE_ADC_BIAS, ADC_INIT=0, cut_frequency=DC_VOLTAGE_ADC_CUT_FREQ}
      mask DialogControl DescGroupVar Prompt: Voltage Sample ADC Model
      mask DialogControl DescTextVar Prompt: This is a ideal Voltage Measurement Module.
      mask DialogControl Control2 Prompt: ADC(p.u.) = (real_voltage * ADC_GAIN + ADC_BIAS)/ADC_REFERENCE
      mask DialogControl Control11 Prompt: GMP CTL Simulink Utilities: virtual peripherals
      mask DialogControl ParameterGroupVar Prompt: Parameters:
      mask DialogControl Control4 Prompt: ADC Voltage Gain (Scale Factor):
      mask DialogControl Control5 Prompt: ADC resolution:
      mask DialogControl Control6 Prompt: ADC reference Voltage(V)
      mask DialogControl Control8 Prompt: ADC Bias Voltage(V)
      mask DialogControl Control7 Prompt: ADC Initial Voltage Output (V):
      mask DialogControl Control9 Prompt: Voltage Filter cut frequency (Hz):
      mask DialogControl Control10 Prompt: Generally, this value less than switch frequency / 10, greater than motor normal frequency * 3
  DC/AC Half Bridge1 : gmp_peripheral_utilities/Single Phase Half Bridge (Duty Model)  fswitch=fswitch  CMP_MAX=CMP_MAX  Deadband_Upper=Deadband_Upper  Deadband_Lower=Deadband_Lower  Deadband_us=NaN  phase_shift=phase_shift  R_mosfet_on=R_mosfet_on  Lon=Lon  Rd=Rd  Vf=Vf  Rs=Rs  Cs=Cs
      settings: SourceProductName=Virtual Peripheral Utilities
  DC/AC Half Bridge2 : gmp_peripheral_utilities/Single Phase Half Bridge (Duty Model)  fswitch=fswitch  CMP_MAX=CMP_MAX  Deadband_Upper=Deadband_Upper  Deadband_Lower=Deadband_Lower  Deadband_us=NaN  phase_shift=phase_shift  R_mosfet_on=R_mosfet_on  Lon=Lon  Rd=Rd  Vf=Vf  Rs=Rs  Cs=Cs
      settings: SourceProductName=Virtual Peripheral Utilities
  Demux : Demux  Outputs=2
  Grid_Current_Sensor : spsSeriesRLCBranchLib/Series RLC Branch  LConnTagsString=__new0  RConnTagsString=__new0  BranchType=R  Resistance=GRID_CURRENT_SENSOR_R  Inductance=1e-3  SetiL0=off  InitialCurrent=0  Capacitance=1e-6  Setx0=off  InitialVoltage=0  Measurements=None
  Ideal Inductor Current Measurement Module（ADC - Current） : Subsystem  AncestorBlock=peripheral_utilities/Ideal Current Measurement Module（ADC - Current）  mask{ADC_GAIN=AC_Current_Gain, ADC_BIT=ADC_Resolution, ADC_REFERENCE=AC_CURRENT_ADC_REFERENCE, ADC_BIAS=AC_CURRENT_ADC_BIAS, ADC_INIT=AC_CURRENT_ADC_INIT}
      mask DialogControl DescGroupVar Prompt: Current Sample ADC Model 1
      mask DialogControl DescTextVar Prompt: This is a ideal Current Measurement Module. This module enable a bias and a gain, and finally output a ADC result.
      mask DialogControl Control8 Prompt: ADC(p.u.) = (real_current * ADC_GAIN + ADC_BIAS)/ADC_REFERENCE
      mask DialogControl Control9 Prompt: GMP CTL Simulink Utilities: virtual peripherals
      mask DialogControl ParameterGroupVar Prompt: 参数
      mask DialogControl Control7 Prompt: ADC Current Gain (Scale Factor):
      mask DialogControl Control2 Prompt: ADC resolution:
      mask DialogControl Control4 Prompt: ADC reference Current(A), ADC full scale current (when gain = 1)
      mask DialogControl Control5 Prompt: ADC Bias Current(A)
      mask DialogControl Control6 Prompt: ADC initial Current Output(A)
  Input_C : spsSeriesRLCBranchLib/Series RLC Branch  LConnTagsString=__new0  RConnTagsString=__new0  BranchType=RC  Resistance=DC_CAP_ESR  Inductance=1e-3  SetiL0=off  InitialCurrent=0  Capacitance=680e-6  Setx0=off  InitialVoltage=0  Measurements=None
  SINV_Current_Sensor : spsSeriesRLCBranchLib/Series RLC Branch  LConnTagsString=__new0  RConnTagsString=__new0  BranchType=R  Resistance=CAP_CURRENT_SENSOR_R  Inductance=1e-3  SetiL0=off  InitialCurrent=0  Capacitance=1e-6  Setx0=off  InitialVoltage=0  Measurements=None
  SINV_DC_BUS_Current_Sensor : spsSeriesRLCBranchLib/Series RLC Branch  LConnTagsString=__new0  RConnTagsString=__new0  BranchType=R  Resistance=DC_BUS_CURRENT_SENSOR_R  Inductance=1e-3  SetiL0=off  InitialCurrent=0  Capacitance=1e-6  Setx0=off  InitialVoltage=0  Measurements=None
  SINV_Filter_C : spsSeriesRLCBranchLib/Series RLC Branch  LConnTagsString=__new0  RConnTagsString=__new0  BranchType=RC  Resistance=ACF_C_ESR  Inductance=1e-3  SetiL0=off  InitialCurrent=0  Capacitance=10e-6  Setx0=off  InitialVoltage=0  Measurements=None
  SINV_Filter_L : spsSeriesRLCBranchLib/Series RLC Branch  LConnTagsString=__new0  RConnTagsString=__new0  BranchType=RL  Resistance=ACF_L_ESR  Inductance=680e-6  SetiL0=off  InitialCurrent=0  Capacitance=1e-6  Setx0=off  InitialVoltage=0  Measurements=None
  Scope{,1..2,8..17} (13 alike) : Scope
  Terminator3 : Terminator
  Voltage Measurement : spsVoltageMeasurementLib/Voltage Measurement  PhasorSimulation=off  OutputType=Complex  PSBequivalent=0
  DC_BUS+ : PMIOPort  Side=Left
  DC_BUS- : PMIOPort  Port=2  Side=Left
  AC_BUS_L : PMIOPort  Port=3  Side=Right
  AC_BUS_N : PMIOPort  Port=4  Side=Right
  ADC Port : Outport
  Trig : Outport  Port=2
  tag scope: VDC=global
  wires:
  DC/AC Half Bridge2/1 -> Ideal Inductor Current Measurement Module（ADC - Current）/1(Sample Trigger), [SampleTrig]
  [BPWM2] -> DC/AC Half Bridge2/2
  AC bus Voltage Measurement Module/2(Scope View (p.u.)) -> Scope8/1
  AC bus Voltage Measurement Module/3(Sample & Hold View) -> Scope9/1
  [EnableTag] -> DC/AC Half Bridge2/1
  DC/AC Half Bridge1/1 -> Terminator3/1
  [SampleTrig] -> DC bus Voltage Measurement Module/1(Sample Trigger)
  Capactor Current Measurement Module/3(Sample & Hold View) -> Scope11/1
  [EnableTag] -> DC/AC Half Bridge1/1
  [SampleTrig] -> Capactor Current Measurement Module/1(Sample Trigger)
  [SampleTrig] -> AC bus Voltage Measurement Module/1(Sample Trigger)
  Capactor Current Measurement Module/2(Scope View (p.u.)) -> Scope10/1
  Capactor Current Measurement Module/1(ADC OUT) -> [Sinv_IC]
  AC bus Voltage Measurement Module/1(ADC OUT) -> [Sinv_VC]
  Ideal Inductor Current Measurement Module（ADC - Current）/3(Sample & Hold View) -> Scope13/1
  DC Bus Current Measurement Module/2(Scope View (p.u.)) -> Scope16/1
  Ideal Inductor Current Measurement Module（ADC - Current）/1(ADC OUT) -> [Sinv_IL]
  Ideal Inductor Current Measurement Module（ADC - Current）/2(Scope View (p.u.)) -> Scope12/1
  DC bus Voltage Measurement Module/2(Scope View (p.u.)) -> Scope14/1
  DC Bus Current Measurement Module/3(Sample & Hold View) -> Scope17/1
  [BPWM1] -> DC/AC Half Bridge1/2
  DC bus Voltage Measurement Module/3(Sample & Hold View) -> [VDC], Scope15/1
  [SampleTrig] -> DC Bus Current Measurement Module/1(Sample Trigger)
  DC bus Voltage Measurement Module/1(ADC OUT) -> [Sinv_VDC]
  DC Bus Current Measurement Module/1(ADC OUT) -> [Sinv_IDC]
  Enable/1 -> [EnableTag]
  PWM CMP/1 -> Demux/1
  Demux/1 -> [BPWM1]
  Demux/2 -> [BPWM2]
  [Sinv_VDC] -> Bus Creator/3
  [Sinv_IDC] -> Bus Creator/2
  [Sinv_IL] -> Bus Creator/1
  [Sinv_IC] -> Bus Creator/4
  [Sinv_VC] -> Bus Creator/5
  Bus Creator/1 -> ADC Port/1
  [SampleTrig] -> Trig/1
  [SampleTrig] -> Capactor Current Measurement Module1/1(Sample Trigger)
  Capactor Current Measurement Module1/1(ADC OUT) -> [Sinv_IG]
  Capactor Current Measurement Module1/2(Scope View (p.u.)) -> Scope1/1
  Capactor Current Measurement Module1/3(Sample & Hold View) -> Scope2/1
  [Sinv_IG] -> Bus Creator/6
  Voltage Measurement/1 -> Scope/1
  connections:
  SINV_Filter_C/LConn1 -- AC_BUS_L/RConn1 -- AC bus Voltage Measurement Module/LConn1 -- SINV_Filter_L/RConn1
  SINV_DC_BUS_Current_Sensor/RConn1 -- DC Bus Current Measurement Module/LConn2 -- Input_C/RConn1 -- DC_BUS-/RConn1
  DC/AC Half Bridge2/RConn2 -- DC bus Voltage Measurement Module/LConn2 -- DC Bus Current Measurement Module/LConn1 -- SINV_DC_BUS_Current_Sensor/LConn1 -- DC/AC Half Bridge1/RConn2
  Capactor Current Measurement Module/LConn1 -- SINV_Filter_C/RConn1 -- SINV_Current_Sensor/LConn1
  Grid_Current_Sensor/LConn1 -- Capactor Current Measurement Module1/LConn1 -- AC_BUS_N/RConn1
  Input_C/LConn1 -- DC_BUS+/RConn1 -- DC/AC Half Bridge1/LConn1 -- DC/AC Half Bridge2/LConn1 -- DC bus Voltage Measurement Module/LConn1
  SINV_Filter_L/LConn1 -- Ideal Inductor Current Measurement Module（ADC - Current）/RConn1
  Ideal Inductor Current Measurement Module（ADC - Current）/LConn1 -- Voltage Measurement/LConn1 -- DC/AC Half Bridge2/RConn1
  Capactor Current Measurement Module/LConn2 -- Capactor Current Measurement Module1/LConn2 -- AC bus Voltage Measurement Module/LConn2 -- Voltage Measurement/LConn2 -- Grid_Current_Sensor/RConn1 -- SINV_Current_Sensor/RConn1 -- DC/AC Half Bridge1/RConn1

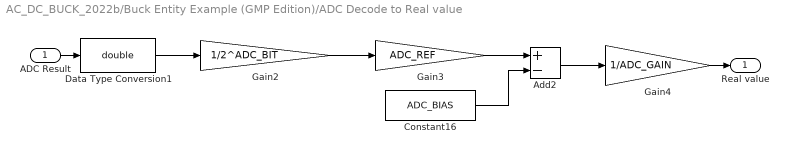
== system AC_DC_BUCK_2022b/Buck Entity Example (GMP Edition)/ADC Decode to Real value ==
  ADC Result : Inport
  Add2 : Sum  Inputs=+-
  Constant16 : Constant  Value=ADC_BIAS
  Data Type Conversion1 : DataTypeConversion  OutDataTypeStr=double  SaturateOnIntegerOverflow=off  RndMeth=Floor
  Gain2 : Gain  Gain=1/2^ADC_BIT
  Gain3 : Gain  Gain=ADC_REF
  Gain4 : Gain  Gain=1/ADC_GAIN
  Real value : Outport
  wires:
  ADC Result/1 -> Data Type Conversion1/1
  Gain2/1 -> Gain3/1
  Constant16/1 -> Add2/2
  Gain4/1 -> Real value/1
  Add2/1 -> Gain4/1
  Gain3/1 -> Add2/1
  Data Type Conversion1/1 -> Gain2/1

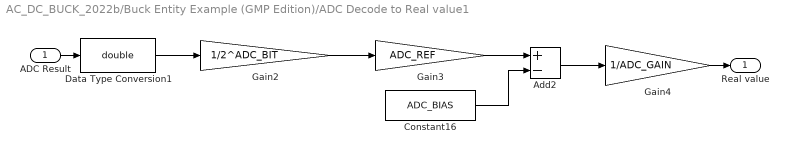
== system AC_DC_BUCK_2022b/Buck Entity Example (GMP Edition)/ADC Decode to Real value1 ==
  ADC Result : Inport
  Add2 : Sum  Inputs=+-
  Constant16 : Constant  Value=ADC_BIAS
  Data Type Conversion1 : DataTypeConversion  OutDataTypeStr=double  SaturateOnIntegerOverflow=off  RndMeth=Floor
  Gain2 : Gain  Gain=1/2^ADC_BIT
  Gain3 : Gain  Gain=ADC_REF
  Gain4 : Gain  Gain=1/ADC_GAIN
  Real value : Outport
  wires:
  ADC Result/1 -> Data Type Conversion1/1
  Gain2/1 -> Gain3/1
  Constant16/1 -> Add2/2
  Gain4/1 -> Real value/1
  Add2/1 -> Gain4/1
  Gain3/1 -> Add2/1
  Data Type Conversion1/1 -> Gain2/1

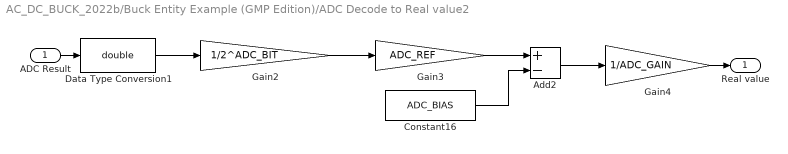
== system AC_DC_BUCK_2022b/Buck Entity Example (GMP Edition)/ADC Decode to Real value2 ==
  ADC Result : Inport
  Add2 : Sum  Inputs=+-
  Constant16 : Constant  Value=ADC_BIAS
  Data Type Conversion1 : DataTypeConversion  OutDataTypeStr=double  SaturateOnIntegerOverflow=off  RndMeth=Floor
  Gain2 : Gain  Gain=1/2^ADC_BIT
  Gain3 : Gain  Gain=ADC_REF
  Gain4 : Gain  Gain=1/ADC_GAIN
  Real value : Outport
  wires:
  ADC Result/1 -> Data Type Conversion1/1
  Gain2/1 -> Gain3/1
  Constant16/1 -> Add2/2
  Gain4/1 -> Real value/1
  Add2/1 -> Gain4/1
  Gain3/1 -> Add2/1
  Data Type Conversion1/1 -> Gain2/1

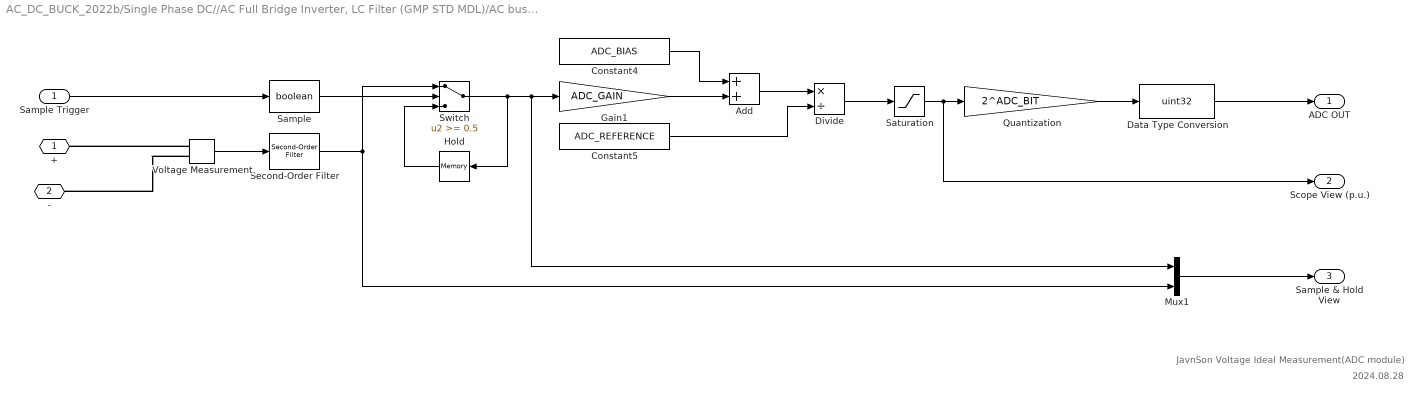
== system AC_DC_BUCK_2022b/Single Phase DC//AC Full Bridge Inverter, LC Filter (GMP STD MDL)/AC bus Voltage Measurement Module ==
  note: 2024.08.28
  note: JavnSon Voltage Ideal Measurement(ADC module)
  Sample Trigger : Inport
  Add : Sum
  Constant4 : Constant  Value=ADC_BIAS
  Constant5 : Constant  Value=ADC_REFERENCE
  Data Type Conversion : DataTypeConversion  OutDataTypeStr=uint32  ConvertRealWorld=Stored Integer (SI)  SaturateOnIntegerOverflow=off  RndMeth=Floor
  Divide : Product  Inputs=*/
  Gain1 : Gain  Gain=ADC_GAIN
  Hold : Memory  InitialCondition=ADC_INIT  LinearizeAsDelay=on
  Mux1 : Mux  Inputs=2
  Quantization : Gain  Gain=2^ADC_BIT
  Sample : DataTypeConversion  OutDataTypeStr=boolean  SaturateOnIntegerOverflow=off  RndMeth=Floor
  Saturation : Saturate  UpperLimit=1  LowerLimit=0
  Second-Order Filter : spsSecondOrderFilterLib/Second-Order Filter  FilterType=Lowpass  Fo=cut_frequency  Zeta=0.707  Ts=0  Initialize=off  Vac_Init="[0,  0,  60]"  Vdc_Init=0  PlotResponse=off  FreqRange=[0, 500, 1]
  Switch : Switch  Threshold=0.5
  Voltage Measurement : spsVoltageMeasurementLib/Voltage Measurement  PhasorSimulation=off  OutputType=Complex  PSBequivalent=0
  + : PMIOPort  Side=Left
  - : PMIOPort  Port=2  Side=Left
  ADC OUT : Outport
  Scope View (p.u.) : Outport  Port=2
  Sample & Hold View : Outport  Port=3
  wires:
  Sample/1 -> Switch/2
  Add/1 -> Divide/1
  Constant5/1 -> Divide/2
  Quantization/1 -> Data Type Conversion/1
  Mux1/1 -> Sample & Hold View/1
  Data Type Conversion/1 -> ADC OUT/1
  Sample Trigger/1 -> Sample/1
  Gain1/1 -> Add/2
  Constant4/1 -> Add/1
  Saturation/1 -> Quantization/1, Scope View (p.u.)/1
  Voltage Measurement/1 -> Second-Order Filter/1
  Divide/1 -> Saturation/1
  Switch/1 -> Gain1/1, Mux1/1, Hold/1
  Hold/1 -> Switch/3
  Second-Order Filter/1 -> Switch/1, Mux1/2
  connections:
  Voltage Measurement/LConn2 -- -/RConn1
  Voltage Measurement/LConn1 -- +/RConn1

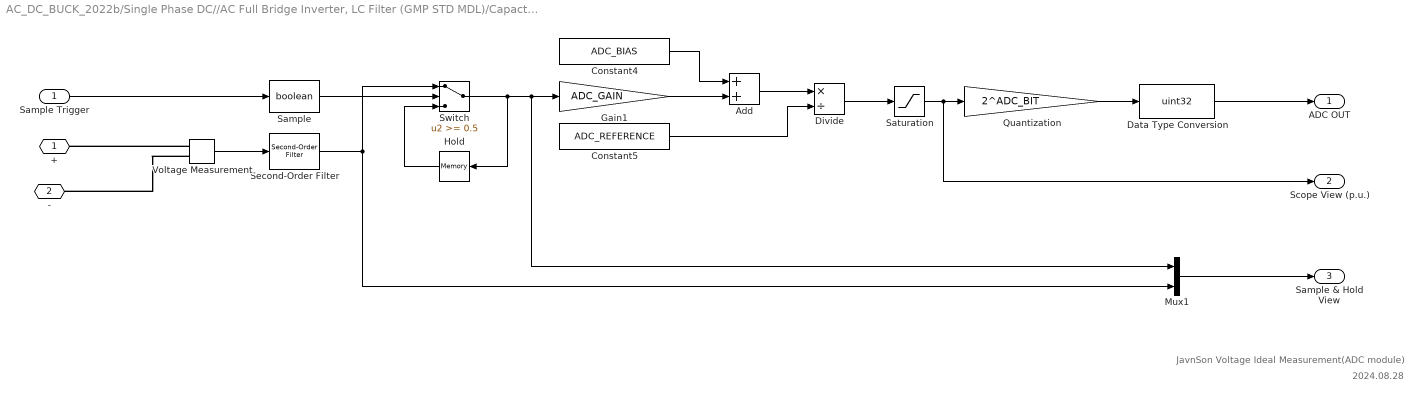
== system AC_DC_BUCK_2022b/Single Phase DC//AC Full Bridge Inverter, LC Filter (GMP STD MDL)/Capactor Current Measurement Module ==
  note: JavnSon Voltage Ideal Measurement(ADC module)
  note: 2024.08.28
  Sample Trigger : Inport
  Add : Sum
  Constant4 : Constant  Value=ADC_BIAS
  Constant5 : Constant  Value=ADC_REFERENCE
  Data Type Conversion : DataTypeConversion  OutDataTypeStr=uint32  ConvertRealWorld=Stored Integer (SI)  SaturateOnIntegerOverflow=off  RndMeth=Floor
  Divide : Product  Inputs=*/
  Gain1 : Gain  Gain=ADC_GAIN
  Hold : Memory  InitialCondition=ADC_INIT  LinearizeAsDelay=on
  Mux1 : Mux  Inputs=2
  Quantization : Gain  Gain=2^ADC_BIT
  Sample : DataTypeConversion  OutDataTypeStr=boolean  SaturateOnIntegerOverflow=off  RndMeth=Floor
  Saturation : Saturate  UpperLimit=1  LowerLimit=0
  Second-Order Filter : spsSecondOrderFilterLib/Second-Order Filter  FilterType=Lowpass  Fo=cut_frequency  Zeta=0.707  Ts=0  Initialize=off  Vac_Init="[0,  0,  60]"  Vdc_Init=0  PlotResponse=off  FreqRange=[0, 500, 1]
  Switch : Switch  Threshold=0.5
  Voltage Measurement : spsVoltageMeasurementLib/Voltage Measurement  PhasorSimulation=off  OutputType=Complex  PSBequivalent=0
  + : PMIOPort  Side=Left
  - : PMIOPort  Port=2  Side=Left
  ADC OUT : Outport
  Scope View (p.u.) : Outport  Port=2
  Sample & Hold View : Outport  Port=3
  wires:
  Second-Order Filter/1 -> Mux1/2, Switch/1
  Hold/1 -> Switch/3
  Switch/1 -> Hold/1, Mux1/1, Gain1/1
  Divide/1 -> Saturation/1
  Voltage Measurement/1 -> Second-Order Filter/1
  Saturation/1 -> Scope View (p.u.)/1, Quantization/1
  Constant4/1 -> Add/1
  Gain1/1 -> Add/2
  Sample Trigger/1 -> Sample/1
  Data Type Conversion/1 -> ADC OUT/1
  Mux1/1 -> Sample & Hold View/1
  Quantization/1 -> Data Type Conversion/1
  Constant5/1 -> Divide/2
  Add/1 -> Divide/1
  Sample/1 -> Switch/2
  connections:
  Voltage Measurement/LConn1 -- +/RConn1
  Voltage Measurement/LConn2 -- -/RConn1
